simulink library "INP_BRK"  (R2024b)
settings: Solver=VariableStepAuto  StartTime=0.0  StopTime=10.0  RelTol=1e-3
libraries: INP_BRK_ManOver x1, INP_BRK_Prep x1
settings Model: Creator=blatak  LastModifiedBy=jmbsp
settings ModelReferenceCC: EnableRefExpFcnMdlSchedulingChecks=on
settings RTWCC: GPUComputeCapability=3.5

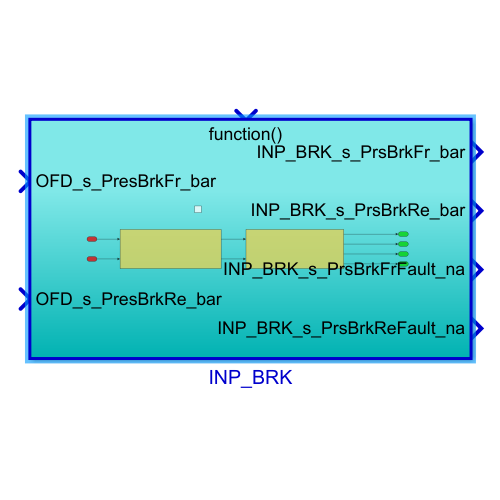
[thumbnail: Simulink's stored preview of the top-level diagram]
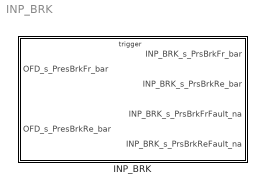
== system INP_BRK ==
  INP_BRK : Subsystem  TreatAsAtomicUnit=on

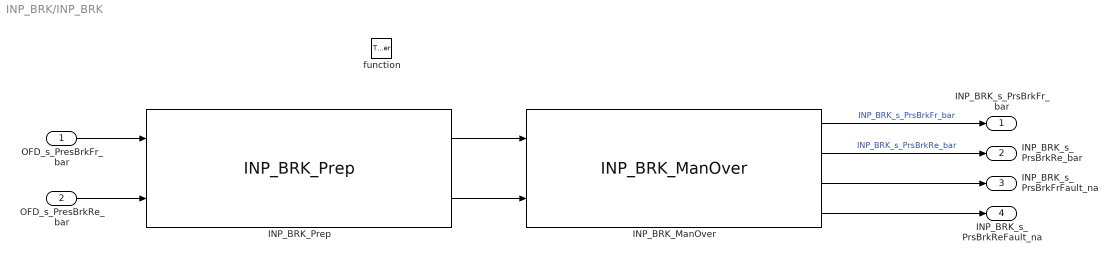
== system INP_BRK/INP_BRK ==
  OFD_s_PresBrkFr_bar : Inport  Description=Front brake pressure - raw measured value
  OFD_s_PresBrkRe_bar : Inport  Description=Rear brake pressure - raw measured value  Port=2
  function : TriggerPort  TriggerType=function-call  VariantControl=(inherit)
  INP_BRK_ManOver : INP_BRK_ManOver/INP_BRK_ManOver  SystemSampleTime=-1  VariantActivationTime=update diagram  AllowFlexibleInterface=on  Latency=0  AutoFrameSizeCalculation=off
  INP_BRK_Prep : INP_BRK_Prep/INP_BRK_Prep  SystemSampleTime=-1  VariantActivationTime=update diagram  AllowFlexibleInterface=on  Latency=0  AutoFrameSizeCalculation=off
  INP_BRK_s_PrsBrkFr_bar : Outport  Description=INP Front brake pressure - value after basic processing, filtering, scale, offset - if necessary
  INP_BRK_s_PrsBrkRe_bar : Outport  Description=INP Rear brake pressure - value after basic processing, filtering, scale, offset - if necessary  Port=2
  INP_BRK_s_PrsBrkFrFault_na : Outport  Port=3
  INP_BRK_s_PrsBrkReFault_na : Outport  Port=4
  wires:
  OFD_s_PresBrkFr_bar/1 -> INP_BRK_Prep/1
  INP_BRK_ManOver/2 -> INP_BRK_s_PrsBrkRe_bar/1  "INP_BRK_s_PrsBrkRe_bar"
  INP_BRK_ManOver/1 -> INP_BRK_s_PrsBrkFr_bar/1  "INP_BRK_s_PrsBrkFr_bar"
  OFD_s_PresBrkRe_bar/1 -> INP_BRK_Prep/2
  INP_BRK_Prep/1 -> INP_BRK_ManOver/1
  INP_BRK_Prep/2 -> INP_BRK_ManOver/2
  INP_BRK_ManOver/3 -> INP_BRK_s_PrsBrkFrFault_na/1
  INP_BRK_ManOver/4 -> INP_BRK_s_PrsBrkReFault_na/1
